simulink model "verify_Wdb2Thb_mdl"  (Simulink 8.2)
settings: Solver=FixedStepDiscrete  StartTime=0  StopTime=1  FixedStep=1  RelTol=1e-3
libraries: carnot x2
settings Model: Creator=drhf  LastModifiedBy=drhf

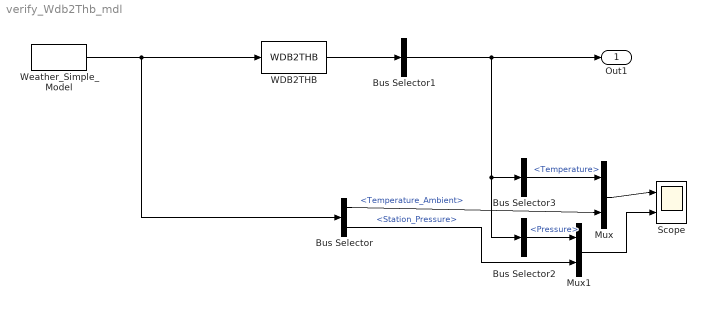
== system verify_Wdb2Thb_mdl ==
  Bus Selector : BusSelector  OutputSignals=Temperature_Ambient,Station_Pressure
  Bus Selector1 : BusSelector  OutputSignals=Temperature,Pressure  OutputAsBus=on
  Bus Selector2 : BusSelector  OutputSignals=Pressure
  Bus Selector3 : BusSelector  OutputSignals=Temperature
  Mux : Mux  Inputs=2
  Mux1 : Mux  Inputs=2
  Scope : Scope  NumInputPorts=2
      settings: YMin=-5~-5  YMax=5~5
  WDB2THB : carnot/Weather/WDB2THB  dia=0.2
  Weather_Simple_Model : carnot/Weather/Weather_Simple_Model  lat=45  Ibn=900  Idg=100  tamb=5  deltaTsky=-6  rh=50  precip="10e-3/24/3600           % 10 mm in 24 h"  cloud=0.125  p=1013e2  vw=1  wdir=270
  Out1 : Outport
  wires:
  Weather_Simple_Model/1 -> Bus Selector/1, WDB2THB/1
  Bus Selector/1 -> Mux/2  "<Temperature_Ambient>"
  WDB2THB/1 -> Bus Selector1/1
  Bus Selector1/1 -> Out1/1, Bus Selector2/1, Bus Selector3/1
  Mux/1 -> Scope/1
  Bus Selector2/1 -> Mux1/1  "<Pressure>"
  Bus Selector/2 -> Mux1/2  "<Station_Pressure>"
  Mux1/1 -> Scope/2
  Bus Selector3/1 -> Mux/1  "<Temperature>"
